simulink model "UNrobot_pro"  (R2021a)
settings: Solver=ode23t  StartTime=0.0  StopTime=t_end  FixedStep=dt  RelTol=1e-3
InitFcn:
  | RPInit
model workspace (MAT data in the model file):
  mapForSim.obsMap = [0 0 0 0 0 0 0 0 0 0 0 0 ... (40000 elements, 200x200)]
  mapForSim.scaleFactor = 5
  mapForSim.simMap = robotics.BinaryOccupancyGrid
  mapForSim.simMap.Grid = [1 1 1 1 1 1 1 1 1 1 1 1 ... (40000 elements, 200x200)]
  mapForSim.simMap.SharedProperties = matlabshared.autonomous.internal.SharedMapProperties
  mapForSim.simMap.SharedProperties.Resolution = 5
  mapForSim.simMap.SharedProperties.GridSize = [200 200]
  mapForSim.simMap.SharedProperties.XLocalLimits = [0 40]
  mapForSim.simMap.SharedProperties.YLocalLimits = [0 40]
  mapForSim.simMap.SharedProperties.XWorldLimits = [0 40]
  mapForSim.simMap.SharedProperties.YWorldLimits = [0 40]
  mapForSim.simMap.SharedProperties.Width = 40
  mapForSim.simMap.SharedProperties.Height = 40
  mapForSim.simMap.SharedProperties.LocalOriginInWorldInternal = [0 0]
  mapForSim.simMap.LayerName = 'binaryLayer'
  mapForSim.simMap.Index = matlabshared.autonomous.internal.CircularBufferIndex
  mapForSim.simMap.Index.Head = [1 1]
  mapForSim.simMap.Index.Size = [200 200]
  mapForSim.simMap.Index.NewRegions = [0 0 0 0]
  mapForSim.simMap.Index.DropEntireMap = 0
  mapForSim.simMap.Index.DropTwoRegions = [0 0]
  mapForSim.simMap.Buffer = matlabshared.autonomous.internal.CircularBuffer
  mapForSim.simMap.Buffer.ConstVal = 0
  mapForSim.simMap.Buffer.DataType = 'logical'
  mapForSim.simMap.Buffer.Index = matlabshared.autonomous.internal.CircularBufferIndex
  mapForSim.simMap.Buffer.Index.Head = [1 1]
  mapForSim.simMap.Buffer.Index.Size = [200 200]
  mapForSim.simMap.Buffer.Index.NewRegions = [0 0 0 0]
  mapForSim.simMap.Buffer.Index.DropEntireMap = 0
  mapForSim.simMap.Buffer.Index.DropTwoRegions = [0 0]
  mapForSim.simMap.Buffer.Buffer = [1 1 1 1 1 1 1 1 1 1 1 1 ... (40000 elements, 200x200)]
  mapForSim.simMap.Buffer.BufferSize = [200 200 1]
  mapForSim.simMap.DefaultValueInternal = 0
  mapForSim.simMap.DataSize = [200 200]
  mapForSim.simMap.GridLocationInWorld = [0 0]
  mapForSim.simMap.GridOriginInLocal = [0 0]
  mapForSim.simMap.LocalOriginInWorld = [0 0]
  mapForSim.simMap.Resolution = 5
  mapForSim.simMap.GridSize = [200 200]
  mapForSim.simMap.XLocalLimits = [0 40]
  mapForSim.simMap.YLocalLimits = [0 40]
  mapForSim.simMap.XWorldLimits = [0 40]
  mapForSim.simMap.YWorldLimits = [0 40]
  mapForSim.simMap.Width = 40
  mapForSim.simMap.Height = 40
  mapForSim.simMap.LocalOriginInWorldInternal = [0 0]
  occGrid = robotics.BinaryOccupancyGrid
  occGrid.Grid = [1 1 1 1 1 1 1 1 1 1 1 1 ... (40000 elements, 200x200)]
  occGrid.SharedProperties = matlabshared.autonomous.internal.SharedMapProperties
  occGrid.SharedProperties.Resolution = 5
  occGrid.SharedProperties.GridSize = [200 200]
  occGrid.SharedProperties.XLocalLimits = [0 40]
  occGrid.SharedProperties.YLocalLimits = [0 40]
  occGrid.SharedProperties.XWorldLimits = [0 40]
  occGrid.SharedProperties.YWorldLimits = [0 40]
  occGrid.SharedProperties.Width = 40
  occGrid.SharedProperties.Height = 40
  occGrid.SharedProperties.LocalOriginInWorldInternal = [0 0]
  occGrid.LayerName = 'binaryLayer'
  occGrid.Index = matlabshared.autonomous.internal.CircularBufferIndex
  occGrid.Index.Head = [1 1]
  occGrid.Index.Size = [200 200]
  occGrid.Index.NewRegions = [0 0 0 0]
  occGrid.Index.DropEntireMap = 0
  occGrid.Index.DropTwoRegions = [0 0]
  occGrid.Buffer = matlabshared.autonomous.internal.CircularBuffer
  occGrid.Buffer.ConstVal = 0
  occGrid.Buffer.DataType = 'logical'
  occGrid.Buffer.Index = matlabshared.autonomous.internal.CircularBufferIndex
  occGrid.Buffer.Index.Head = [1 1]
  occGrid.Buffer.Index.Size = [200 200]
  occGrid.Buffer.Index.NewRegions = [0 0 0 0]
  occGrid.Buffer.Index.DropEntireMap = 0
  occGrid.Buffer.Index.DropTwoRegions = [0 0]
  occGrid.Buffer.Buffer = [1 1 1 1 1 1 1 1 1 1 1 1 ... (40000 elements, 200x200)]
  occGrid.Buffer.BufferSize = [200 200 1]
  occGrid.DefaultValueInternal = 0
  occGrid.DataSize = [200 200]
  occGrid.GridLocationInWorld = [0 0]
  occGrid.GridOriginInLocal = [0 0]
  occGrid.LocalOriginInWorld = [0 0]
  occGrid.Resolution = 5
  occGrid.GridSize = [200 200]
  occGrid.XLocalLimits = [0 40]
  occGrid.YLocalLimits = [0 40]
  occGrid.XWorldLimits = [0 40]
  occGrid.YWorldLimits = [0 40]
  occGrid.Width = 40
  occGrid.Height = 40
  occGrid.LocalOriginInWorldInternal = [0 0]
values from neighbouring files (symbols this model uses):
  obstacles = eval(get_param(block,'obstacles'))    [RPInit.m]    (also in setup.m = csvread('obstacles2.csv'))
  Ts = 0.1    [setup.m]
undefined symbols (not defined in the file or in its folder): FloorSurface, Ref, RobotSurface, T_max, Wall1Surface, Wall2Surface, Wall3Surface, Wall4Surface, WallSurface, X, Y, Z
libraries: sm_lib x52, nesl_utility x18, RP_Simulator_Components x16, RoboticsPlayground x9, simulink x6
(part 1 of 3)
settings Model: EnablePacing=on  Creator=josea  LastModifiedBy=Sebastian
settings SolverCC: AlgebraicLoopSolver=TrustRegion
settings DataIOCC: ReturnWorkspaceOutputs=off
settings DebuggingCC: UnconnectedLineMsg=none  SFMachineParentedDataDiag=warning  ArithmeticOperatorsInVariantConditions=warning
settings SFSimCC: SimUseLocalCustomCode=off  CustomCodeUndefinedFunction=UseInterfaceOnly
settings RTWCC: RTWUseLocalCustomCode=off
settings DiagnosticsConfigSet: SimMechanicsRigidlyBoundBlock=none
settings ExplorerConfigSet: InternalSimMechanicsExplorerSettings="<ExplorerConfiguration><canonicalview>default</canonicalview><AnimationSetting><BasePlaybackSpeed>1.0</BasePlaybackSpeed><PlaybackSpeedFactor>1.0</PlaybackSpeedFactor></AnimationSetting><TilePanel><TileInfo><Tiles Columns=\"2\" Count=\"3\" Rows=\"2\"><Column Weight=\"0.4996\"/><Column Weight=\"0.5004\"/><Row Weight=\"0.4995\"/><Row Weight=\"0.5005\"/><Tile Height=\"1\" Width=\"2\" X=\"0\" Y=\"0\"/><Tile Height=\"1\" Width=\"1\" X=\"0\" Y=\"1\"/><Tile Height=\"1\" Width=\"1\" X=\"1\" Y=\"1\"/></Tiles></TileInfo><SceneInfo><SceneViewer><BGColor><R>0.400000005960464478</R><G>0.400000005960464478</G><B>0.400000005960464478</B></BGColor><Camera><DoPerspective>off</DoPerspective><Position><X>42.9310669159878344</X><Y>-10.3897658506810977</Y><Z>43.7453005085714111</Z></Position><Center><X>20.3419761828377759</X><Y>23.2650901944664916</Y><Z>12.1932033045180681</Z></Center><Up><X>-0.363361854461093647</X><Y>0.495671071722158407</Y><Z>0.788846215291930219</Z></Up><ViewLimDist>1</ViewLimDist><YLim>30.3164478917145566</YLim><XLim>117.138200069864226</XLim></Camera></SceneViewer><SceneViewer><BGColor><R>0.400000005960464478</R><G>0.400000005960464478</G><B>0.400000005960464478</B></BGColor><Camera><DoPerspective>on</DoPerspective><Position><X>8.06324715656376156</X><Y>-1.11711218962495051</Y><Z>0.353907143146574898</Z></Position><Center><X>7.7585532943741855</X><Y>-0.164661849531568261</Y><Z>0.353907143146574954</Z></Center><Up><X>5.06422372314121883e-17</X><Y>-4.83127509520006689e-17</Y><Z>1</Z></Up><ViewLimDist>1</ViewLimDist><YLim>0.466307658154998583</YLim><XLim>0.89330132171144927</XLim></Camera></SceneViewer><SceneViewer><BGColor><R>0.400000005960464478</R><G>0.400000005960464478</G><B>0.400000005960464478</B></BGColor><Camera><DoPerspective>off</DoPerspective><Position><X>9.39383108584540416</X><Y>-0.802378430868030179</Y><Z>41.4375460163895966</Z></Position><Center><X>9.39383108584540416</X><Y>-0.802378430868030179</Y><Z>2.33605756749020088</Z></Center><Up><X>0</X><Y>1</Y><Z>-0</Z></Up><ViewLimDist>1</ViewLimDist><YLim>18.9446942541944559</YLim><XLim>36.3365447170614928</XLim></Camera></SceneViewer></SceneInfo></TilePanel><MechEditorPanel><Cameras><Camera><Id>Camera1</Id><Value><Name>RobotView</Name><NativeCamera><PositionTrackingFeature>Obstacle_Environment.Robot.Body.RobotCamera.F</PositionTrackingFeature><CenterTrackingFeature>Obstacle_Environment.Robot.Body.RobotCamera.F</CenterTrackingFeature><UpVectorTrackingFeature>Obstacle_Environment.Robot.Body.RobotCamera.F</UpVectorTrackingFeature><CenterTrackingOrigin>off</CenterTrackingOrigin><CenterTrackingDirection>+X</CenterTrackingDirection><UpVectorTrackingDirection>+Z</UpVectorTrackingDirection></NativeCamera></Value></Camera></Cameras><GfxPanelCameraMap><MapElement CameraMLId=\"Camera1\" GfxPanelIndex=\"1\"/></GfxPanelCameraMap><VideoCreator><PlaybackSpeedRatio>1.0</PlaybackSpeedRatio><FrameRate>30</FrameRate><VideoFormat>MPEG-4</VideoFormat><FrameSize>[1920 1080]</FrameSize></VideoCreator></MechEditorPanel></ExplorerConfiguration>"

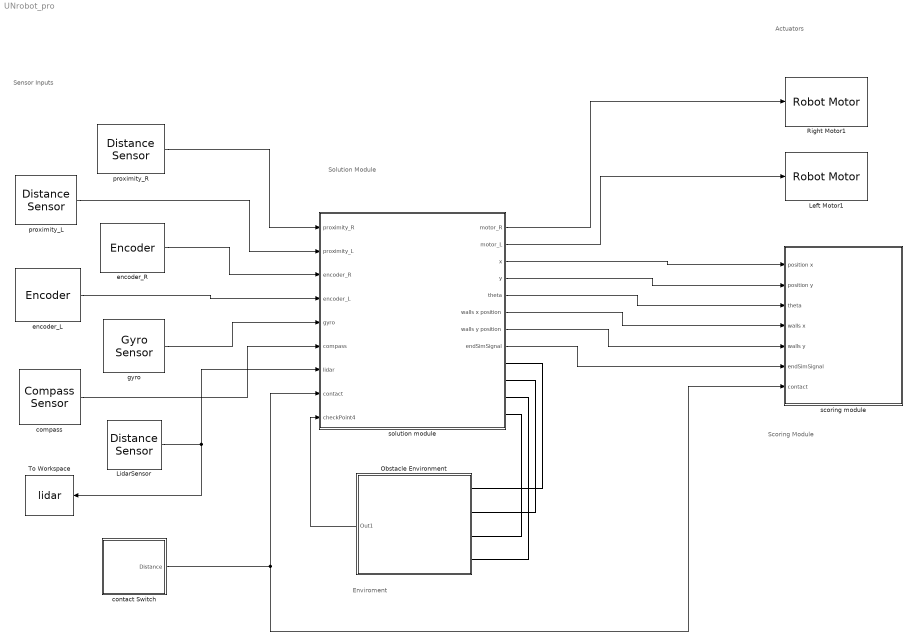
== system UNrobot_pro ==
  note: Solution Module
  note: Actuators
  note: Scoring Module
  note: Sensor Inputs
  note: Enviroment
  Left Motor1 : RoboticsPlayground/Basic Sensors and Actuators/Robot Motor  robotId=1  motorChoice=1
      settings: SourceProductName=Robotics Playground
  LidarSensor : RoboticsPlayground/Basic Sensors and Actuators/Distance Sensor  robotId=1  maxSenRange=4  minSenRange=0.02  senRes=0.01  sensOff=[-0.1 0]  sensOffDeg=0  sensorTs=0.1  mask(RP Distance Sensor){}
      link override MATLAB System: scanAngles=linspace(-pi,pi,37)
      settings: SourceProductName=Robotics Playground
      mask Display: image('$imagefile'); % Use "Edit Image" on toolstrip to change.
  Obstacle Environment : Subsystem  mask(RP Obstacle Environment){obstacles=obstacles, arenaLength=40, arenaWidth=40, robotId=1, wheelBase=0.5, wheelRadius=0.1, robotColor=[0.5 0 0], startPose=[0 0]}
      mask prompts: obstacles "Obstacles matrix[nx4] with rectangles with the form [x,y,length,width]"; arenaLength "Length [m]"; arenaWidth "Width [m]"; robotId "Robot ID"; wheelBase "Distance between wheels [m]"; wheelRadius "Wheel radius [m]"; robotColor "Color [R G B]"; startPose "Initial Position X Y [m]"
      mask help:
      | This block contains a virtual environment for a single robot to interact with walls, obstacles and objects. Sensors implemented in the Robotics Playground library can be used to obtain environment information and actuators to interact with the robot behavior.
      |
      | Motor mapping for the robot is as follows:
      |
      | Motor 1 -> Left wheel motor torque
      | Motor 2 -> Right wheel motor torque
      settings: CopyFcn=|
      | set_param(gcs,'InitFcn','RPInit');
      | set_param(gcs,'Solver','ode23t');
      | set_param(gcs, 'EnablePacing', 'on')
      | set_param(gcs, 'PacingRate', 1)
      mask Help: web('obstacle_arena.htm')
      mask DialogControl obsT Prompt: Obstacle settings
      mask DialogControl Container19 Prompt: Set Obstacles Interactively
      mask DialogControl Control2 Prompt: Set Obstacles
      mask DialogControl Control2 Callback: setObstaclesUI(gcb)
      mask DialogControl Container6 Prompt: Arena settings
      mask DialogControl Container4 Prompt: Robot settings
      mask Display:
      | color('white');
      | plot([100,100,100,100]*1,[100,100,100,100]*1);
      | plot([100,100,100,100]*0,[100,100,100,100]*0);
      | image('ObstacleEnv.PNG')
      | color('blue');
      | id=eval(get_param(gcb,'robotId'));
      | text(99, 92, ['Robot ID: ' num2str(id)], 'horizontalAlignment', 'right');
  Right Motor1 : RoboticsPlayground/Basic Sensors and Actuators/Robot Motor  robotId=1  motorChoice=2
      settings: SourceProductName=Robotics Playground
  To Workspace : ToWorkspace  VariableName=lidar  SaveFormat=Structure  SampleTime=-1
  "compass " : RoboticsPlayground/Basic Sensors and Actuators/Compass Sensor  robotId=1  sensorTs=0.01
      settings: SourceProductName=Robotics Playground
  contact Switch : Subsystem  AncestorBlock=RoboticsPlayground/Basic Sensors and Actuators/Contact Switch  mask(RP Contact Switch){robotId=1, trigDist=0.251, sensOff=[0 0], sensOffDeg=0, sensorTs=0.1}
      mask prompts: robotId "Robot ID"; trigDist "Trigger Distance [m]"; sensOff "Sensor Position Offset X Y [m]"; sensOffDeg "Sensor Orientation Offset [deg]"; sensorTs "Sensor sample time [s]"
      mask help:
      | This block outputs 1 if the sensor comes in close proximity to a wall or obstacle. Otherwise it outputs zero. The proximity at which the sensor is triggered can be set through the mask using the "Trigger Distance" field. Default values can also be used.
      |
      | Sensor position and orientation offsets are with respect to the robot center.
      mask init:
      | ID=get_param(gcb,'robotId');
      | 
      | set_param([gcb '/xPose'],'GotoTag',['R' ID 'xPose']);
      | set_param([gcb '/yPose'],'GotoTag',['R' ID 'yPose']);
      | set_param([gcb '/tPose'],'GotoTag',['R' ID 'tPose']);
      mask Help: web('contact_switch.htm')
      mask DialogControl senCont Prompt: Sensor Characteristics
      mask Display:
      | color('white');
      | plot([100,100,100,100]*1,[100,100,100,100]*1);
      | plot([100,100,100,100]*0,[100,100,100,100]*0);
      | image('ContactSwitch.png','center')
      | color('blue');
      | id=eval(get_param(gcb,'robotId'));
      | text(99, 92, ['Robot ID: ' num2str(id)], 'horizontalAlignment', 'right');
  encoder_L : RoboticsPlayground/Basic Sensors and Actuators/Encoder  robotId=1  motorChoice=1  rstChoice=No reset  ticks=encoder_ticks  detectDir=on  sensorTs=0.1
      settings: SourceProductName=Robotics Playground
  encoder_R : RoboticsPlayground/Basic Sensors and Actuators/Encoder  robotId=1  motorChoice=2  rstChoice=No reset  ticks=encoder_ticks  detectDir=on  sensorTs=0.1
      settings: SourceProductName=Robotics Playground
  "gyro " : RoboticsPlayground/Basic Sensors and Actuators/Gyro Sensor  robotId=1  sensor=Body Center  sensorTs=0.01
      settings: SourceProductName=Robotics Playground
  proximity_L : RoboticsPlayground/Basic Sensors and Actuators/Distance Sensor  robotId=1  maxSenRange=2  minSenRange=0.02  senRes=0.01  sensOff=P_L  sensOffDeg=45  sensorTs=0.1
      settings: SourceProductName=Robotics Playground
  proximity_R : RoboticsPlayground/Basic Sensors and Actuators/Distance Sensor  robotId=1  maxSenRange=2  minSenRange=0.02  senRes=0.01  sensOff=P_R  sensOffDeg=-45  sensorTs=0.1  mask(RP Distance Sensor){}
      settings: SourceProductName=Robotics Playground
  scoring module : Subsystem
  solution module : Subsystem
  wires:
  proximity_R/1 -> solution module/1(proximity_R)
  proximity_L/1 -> solution module/2(proximity_L)
  encoder_R/1 -> solution module/3(encoder_R)
  encoder_L/1 -> solution module/4(encoder_L)
  "gyro "/1 -> solution module/5(gyro)
  "compass "/1 -> solution module/6(compass)
  contact Switch/1(Distance) -> solution module/8(contact), scoring module/7(contact)
  solution module/2(motor_L) -> Left Motor1/1
  solution module/1(motor_R) -> Right Motor1/1
  solution module/3(x) -> scoring module/1(position x)
  solution module/4(y) -> scoring module/2(position y)
  solution module/5(theta) -> scoring module/3(theta)
  Obstacle Environment/1(Out1) -> solution module/9(checkPoint4)
  LidarSensor/1 -> To Workspace/1, solution module/7(lidar)
  solution module/6(walls x position) -> scoring module/4(walls x)
  solution module/7(walls y position) -> scoring module/5(walls y)
  solution module/8(endSimSignal) -> scoring module/6(endSimSignal)
  connections:
  Obstacle Environment/LConn4 -- solution module/RConn3
  Obstacle Environment/LConn1 -- solution module/RConn1
  Obstacle Environment/LConn2 -- solution module/RConn2
  Obstacle Environment/LConn3 -- solution module/RConn4

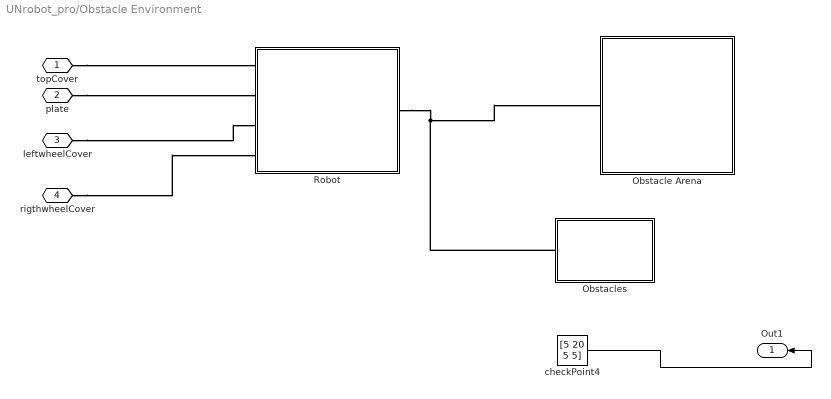
== system UNrobot_pro/Obstacle Environment ==
  Obstacle Arena : Subsystem  AncestorBlock=RP_Simulator_Components/Obstacle Arena  mask(RP Grid Arena){length=arenaLength, width=arenaWidth, robotRadius=wheelBase/2, checkPoint4=[5 20 5 5]}
      mask prompts: length "Arena length [m]"; width "Arena width [m]"; robotRadius "Robot Radius [m]"; checkPoint4 "check point 4 position [x,y, Length Width]"
      mask help: This block is an arena for robots to operate within. This arena implements contact between one robot and the walls and also introduces a floor grid for better visualization. Connect to other robots within the library using the corresponding "Robot" and "Ref" ports.
      mask DialogControl Container5 Prompt: Arena dimensions
      mask Display:
      | image('ObstacleArena.PNG')
      | port_label('Lconn',1,'RP-Bus')
  Obstacles : Subsystem
  Robot : Subsystem  AncestorBlock=RP_Simulator_Components/Contact Tank Robot  mask(RP Contact Tank Robot){robotId=robotId, wheelRadius=wheelRadius, wheelBase=wheelBase, wheelThickness=0.025, chassisThickness=0.05, startPose=startPose, choice=off, sensorTs=0.05, wheelMass=0.2, chassisMass=0.5, maxWheelTorque=T_max, floorSize=[arenaLength arenaWidth], wheelColor=[0.25 0.25 0.25], chassisColor=robotColor}
      mask prompts: robotId "Robot ID"; wheelRadius "Wheel Radius [m]"; wheelBase "Wheelbase [m]"; wheelThickness "Wheel Thickness [m]"; chassisThickness "Chassis Thickness [m]"; startPose "Start Position [m]"; choice "Reverse Start Position"; sensorTs "Sensor sample time [s]"; wheelMass "Wheel Mass [kg]"; chassisMass "Chassis Mass [kg]"; maxWheelTorque "Maximum wheel torque [N*m]"; floorSize "Floor Dimensions [m]"; wheelColor "Wheel Color"; chassisColor "Chassis Color"
      mask help:
      | This robot implements contact between the robot wheels and the floor of an arena. The stck-slip friction implemented using contact force libraries makes the robot behavior more realistic. The inputs to the robot are now motor torque, which is set using the Robotics Playground Motor blocks. The motor mappings are as follows:
      |
      | Motor 1 -> Left wheel motor torque
      | Motor 2 -> Right wheel motor torque
      mask init:
      | block=gcb;
      | ID=num2str(eval(get_param(block,'robotId')));
      | 
      | set_param([block '/motor1t'],'GotoTag',['R' ID 'motor1t']);
      | set_param([block '/motor2t'],'GotoTag',['R' ID 'motor2t']);
      | set_param([block '/motor1q'],'GotoTag',['R' ID 'motor1q']);
      | set_param([block '/motor1w'],'GotoTag',['R' ID 'motor1w']);
      | set_param([block '/motor2q'],'GotoTag',['R' ID 'motor2q']);
      | set_param([block '/motor2w'],'GotoTag',['R' ID 'motor2w']);
      | set_param([block '/xPose'],'GotoTag',['R' ID 'xPose']);
      | set_param([block '/yPose'],'GotoTag',['R' ID 'yPose']);
      | set_param([block '/tPose'],'GotoTag',['R' ID 'tPose']);
      | set_param([block '/tRate'],'GotoTag',['R' ID 'tRate']);
      | set_param([block '/tAngle'],'GotoTag',['R' ID 'tAngle']);
      | 
      | % Add sensor visuals
      | 
      | addSensors(block,eval(ID));
      mask DialogControl KinContainer Prompt: Kinematics
      mask DialogControl DynamicsContainer Prompt: Dynamics
      mask DialogControl AppearanceContainer Prompt: Appearance
      mask Display:
      | image('discRobot.PNG')
      | port_label('Rconn',1,'RP-Bus')
  checkPoint4 : Constant  Value=[5 20 5 5]
  topCover : PMIOPort  Side=Left
  plate : PMIOPort  Port=2  Side=Left
  leftwheelCover : PMIOPort  Port=3  Side=Left
  rigthwheelCover : PMIOPort  Port=4  Side=Left
  Out1 : Outport
  wires:
  checkPoint4/1 -> Out1/1
  connections:
  Obstacles/LConn1 -- Robot/RConn1 -- Obstacle Arena/LConn1
  topCover/RConn1 -- Robot/LConn1
  plate/RConn1 -- Robot/LConn2
  leftwheelCover/RConn1 -- Robot/LConn3
  rigthwheelCover/RConn1 -- Robot/LConn4

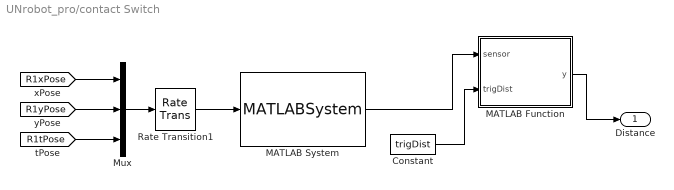
== system UNrobot_pro/contact Switch ==
  Constant : Constant  Value=trigDist
  MATLAB Function : MATLAB Function  TreatAsAtomicUnit=on
  MATLAB System : MATLABSystem  System=LidarSensorRP  mapName=occGrid  sensorOffset=sensOff  scanAngles=linspace(-pi,pi,50)  maxRange=trigDist+1
      mask Type: LidarSensorRP
      mask Display:
      | disp(['Lidar' char(10) 'Sensor']);
      | port_label('input',1,'pose');
      | port_label('output',1,'ranges');
  Mux : Mux  Inputs=3
  Rate Transition1 : RateTransition  OutPortSampleTime=sensorTs
  Distance : Outport  VectorParamsAs1DForOutWhenUnconnected=off
  wires:
  Rate Transition1/1 -> MATLAB System/1
  MATLAB Function/1(y) -> Distance/1
  Constant/1 -> MATLAB Function/2(trigDist)
  MATLAB System/1 -> MATLAB Function/1(sensor)
  [R1xPose] -> Mux/1
  [R1yPose] -> Mux/2
  [R1tPose] -> Mux/3
  Mux/1 -> Rate Transition1/1

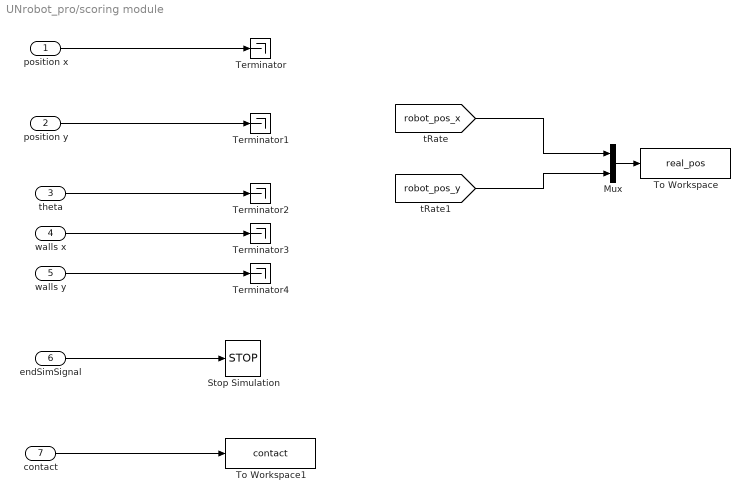
== system UNrobot_pro/scoring module ==
  position x : Inport
  position y : Inport  Port=2
  theta : Inport  Port=3
  walls x : Inport  Port=4
  walls y : Inport  Port=5
  endSimSignal : Inport  Port=6
  contact : Inport  Port=7
  Mux : Mux  Inputs=2
  Stop Simulation : Stop
  Terminator{,1..4} (5 alike) : Terminator
  To Workspace : ToWorkspace  VariableName=real_pos  SaveFormat=Structure With Time  SampleTime=Ts
  To Workspace1 : ToWorkspace  VariableName=contact  SaveFormat=Structure  SampleTime=Ts
  wires:
  position x/1 -> Terminator/1
  position y/1 -> Terminator1/1
  theta/1 -> Terminator2/1
  [robot_pos_x] -> Mux/1
  [robot_pos_y] -> Mux/2
  Mux/1 -> To Workspace/1
  endSimSignal/1 -> Stop Simulation/1
  contact/1 -> To Workspace1/1
  walls x/1 -> Terminator3/1
  walls y/1 -> Terminator4/1

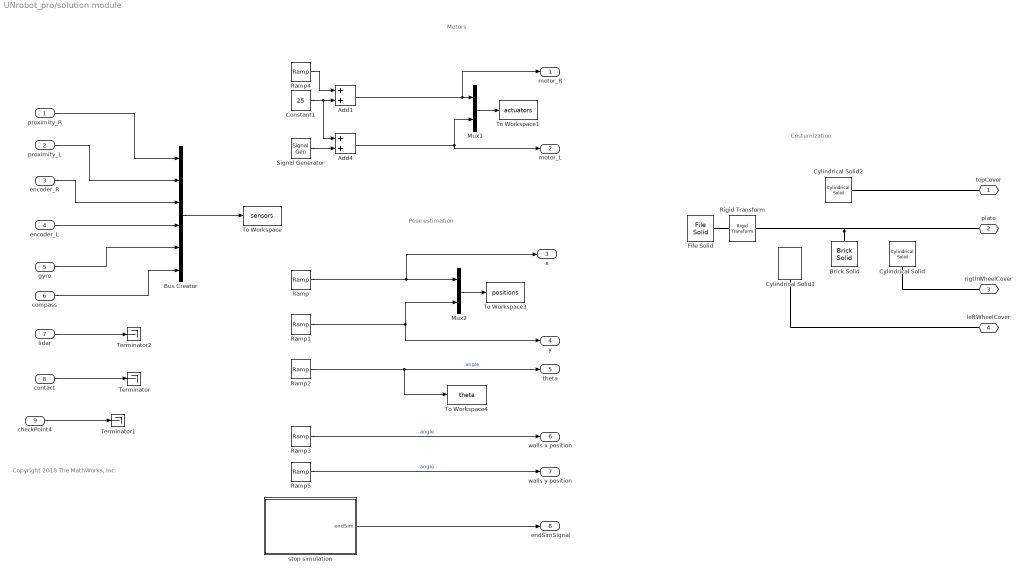
== system UNrobot_pro/solution module ==
  note: Copyright 2018 The MathWorks, Inc.
  note: Pose estimation
  note: Costumization
  note: Motors
  proximity_R : Inport
  proximity_L : Inport  Port=2
  encoder_R : Inport  Port=3
  encoder_L : Inport  Port=4
  gyro : Inport  Port=5
  compass : Inport  Port=6
  lidar : Inport  Port=7
  contact : Inport  Port=8
  checkPoint4 : Inport  Port=9
  Add1 : Sum
  Add4 : Sum
  Brick Solid : sm_lib/Body Elements/Brick Solid  GraphicAmbientColor=[0.15 0.15 0.15 1.0]  BasedOnType=Density  BrickDimensions=[0.1 0.25 0.05]  BrickDimensionUnits=m  CenterOfMass=[0 0 0]  CenterOfMassUnits=m  GraphicDiffuseColor=[ 0 1 0.5]  Density=1000  DensityUnits=kg/m^3  DoExposeReferenceFrame=off  GraphicEmissiveColor=[0.0 0.0 0.0 1.0]  ExportEntireGeometry=off  SerializedFrames=<Frames><Frame><Id>Frame1</Id><Value><Name>F1</Name><Origin><Source>GeometricFeature</Source><FeatureName>+z surface</FeatureName></Origin><PrimaryAxis><DefinedDirection>+Z</DefinedDirection><Source>ReferenceFrame</Source><SourceDirection>+Z</SourceDirection><FeatureName></FeatureName></PrimaryAxis><SecondaryAxis><DefinedDirection>+X</DefinedDirection><Source>ReferenceFrame</Source><SourceDirection>+X</SourceDirection><FeatureName></FeatureName></SecondaryAxis></Value></Frame></Frames>  MarkerShape=Sphere  MarkerSize=10  GraphicType=FromGeometry  InertiaType=PointMass  Mass=0  MassUnits=kg  MomentsOfInertia=[1 1 1]  MomentsOfInertiaUnits=kg*m^2  GraphicOpacity=0.4  ProductsOfInertia=[0 0 0]  ProductsOfInertiaUnits=kg*m^2  GraphicShininess=75  GraphicSpecularColor=[0.5 0.5 0.5 1.0]  GraphicVisPropType=SimpleVisualProperties
  Bus Creator : BusCreator  Inputs=6
  Constant1 : Constant  Value=25
  Cylindrical Solid : sm_lib/Body Elements/Cylindrical Solid  GraphicAmbientColor=[0.15 0.15 0.15 1.0]  BasedOnType=Density  CenterOfMass=[0 0 0]  CenterOfMassUnits=m  GraphicDiffuseColor=[0 1 0.5]  CylinderLength=0.05  CylinderLengthUnits=m  CylinderRadius=0.1  CylinderRadiusUnits=m  Density=1000  DensityUnits=kg/m^3  DoExposeReferenceFrame=off  GraphicEmissiveColor=[0.0 0.0 0.0 1.0]  ExportEntireGeometry=off  SerializedFrames=<Frames><Frame><Id>Frame1</Id><Value><Name>F1</Name><Origin><Source>GeometricFeature</Source><FeatureName>bottom surface</FeatureName></Origin><PrimaryAxis><DefinedDirection>+Z</DefinedDirection><Source>ReferenceFrame</Source><SourceDirection>+Z</SourceDirection><FeatureName></FeatureName></PrimaryAxis><SecondaryAxis><DefinedDirection>+X</DefinedDirection><Source>ReferenceFrame</Source><SourceDirection>+X</SourceDirection><FeatureName></FeatureName></SecondaryAxis></Value></Frame></Frames>  MarkerShape=Sphere  MarkerSize=10  GraphicType=FromGeometry  InertiaType=CalculateFromGeometry  Mass=1  MassUnits=kg  MomentsOfInertia=[1 1 1]  MomentsOfInertiaUnits=kg*m^2  GraphicOpacity=0.1  ProductsOfInertia=[0 0 0]  ProductsOfInertiaUnits=kg*m^2  GraphicShininess=75  GraphicSpecularColor=[0.5 0.5 0.5 1.0]  GraphicVisPropType=SimpleVisualProperties
  Cylindrical Solid1 : sm_lib/Body Elements/Cylindrical Solid  GraphicAmbientColor=[0.15 0.15 0.15 1.0]  BasedOnType=Density  CenterOfMass=[0 0 0]  CenterOfMassUnits=m  GraphicDiffuseColor=[0 1 0.5 ]  CylinderLength=0.05  CylinderLengthUnits=m  CylinderRadius=0.1  CylinderRadiusUnits=m  Density=1000  DensityUnits=kg/m^3  DoExposeReferenceFrame=off  GraphicEmissiveColor=[0.0 0.0 0.0 1.0]  ExportEntireGeometry=off  SerializedFrames=<Frames><Frame><Id>Frame1</Id><Value><Name>F1</Name><Origin><Source>GeometricFeature</Source><FeatureName>bottom surface</FeatureName></Origin><PrimaryAxis><DefinedDirection>+Z</DefinedDirection><Source>ReferenceFrame</Source><SourceDirection>+Z</SourceDirection><FeatureName></FeatureName></PrimaryAxis><SecondaryAxis><DefinedDirection>+X</DefinedDirection><Source>ReferenceFrame</Source><SourceDirection>+X</SourceDirection><FeatureName></FeatureName></SecondaryAxis></Value></Frame></Frames>  MarkerShape=Sphere  MarkerSize=10  GraphicType=FromGeometry  InertiaType=PointMass  Mass=0  MassUnits=kg  MomentsOfInertia=[1 1 1]  MomentsOfInertiaUnits=kg*m^2  GraphicOpacity=0.1  ProductsOfInertia=[0 0 0]  ProductsOfInertiaUnits=kg*m^2  GraphicShininess=75  GraphicSpecularColor=[0.5 0.5 0.5 1.0]  GraphicVisPropType=SimpleVisualProperties
  Cylindrical Solid2 : sm_lib/Body Elements/Cylindrical Solid  GraphicAmbientColor=[0.15 0.15 0.15 1.0]  BasedOnType=Density  CenterOfMass=[0 0 0]  CenterOfMassUnits=m  GraphicDiffuseColor=[0 1 0.5]  CylinderLength=0.5  CylinderLengthUnits=m  CylinderRadius=0.25  CylinderRadiusUnits=m  Density=1000  DensityUnits=kg/m^3  DoExposeReferenceFrame=off  GraphicEmissiveColor=[0.0 0.0 0.0 1.0]  ExportEntireGeometry=off  SerializedFrames=<Frames><Frame><Id>Frame1</Id><Value><Name>F1</Name><Origin><Source>GeometricFeature</Source><FeatureName>bottom surface</FeatureName></Origin><PrimaryAxis><DefinedDirection>+Z</DefinedDirection><Source>ReferenceFrame</Source><SourceDirection>+Z</SourceDirection><FeatureName></FeatureName></PrimaryAxis><SecondaryAxis><DefinedDirection>+X</DefinedDirection><Source>ReferenceFrame</Source><SourceDirection>+X</SourceDirection><FeatureName></FeatureName></SecondaryAxis></Value></Frame></Frames>  MarkerShape=Sphere  MarkerSize=10  GraphicType=FromGeometry  InertiaType=PointMass  Mass=0  MassUnits=kg  MomentsOfInertia=[1 1 1]  MomentsOfInertiaUnits=kg*m^2  GraphicOpacity=0.1  ProductsOfInertia=[0 0 0]  ProductsOfInertiaUnits=kg*m^2  GraphicShininess=75  GraphicSpecularColor=[0.5 0.5 0.5 1.0]  GraphicVisPropType=SimpleVisualProperties
  File Solid : sm_lib/Body Elements/File Solid  ExtGeomFileName=CAD\placa.step  UnitType=FromFile  ExtGeomFileUnits=cm  StepReaderType=HEX  ExportConvexHullGeometry=off  InertiaType=PointMass  Mass=0  MassUnits=kg  CenterOfMass=[0 0 0]  CenterOfMassUnits=m  MomentsOfInertia=[1 1 1]  MomentsOfInertiaUnits=kg*m^2  ProductsOfInertia=[0 0 0]  ProductsOfInertiaUnits=kg*m^2  BasedOnType=DensityFromFile  Density=1000  DensityUnits=kg/m^3  DoExposeReferenceFrame=on  SerializedFrames=<Frames/>  GraphicType=FromGeometry  MarkerShape=Sphere  MarkerSize=10  GraphicVisPropType=SimpleVisualProperties  GraphicDiffuseColor=[1 1 1]  GraphicSpecularColor=[0.5 0.5 0.5 1.0]  GraphicAmbientColor=[0.15 0.15 0.15 1.0]  GraphicEmissiveColor=[0.0 0.0 0.0 1.0]  GraphicShininess=75  GraphicOpacity=1.0
  Mux1 : Mux  Inputs=2
  Mux2 : Mux  Inputs=2
  Ramp{,1..5} (6 alike) : simulink/Sources/Ramp  slope=1  start=0  InitialOutput=0
  Rigid Transform : sm_lib/Frames and Transforms/Rigid Transform  TranslationMethod=None  TranslationStandardOffset=0  TranslationLengthUnit=m  TranslationStandardAxis=+Z  TranslationCartesianOffset=[0 0 0]  TranslationROffset=0  TranslationROffsetUnits=m  TranslationZOffset=0  TranslationZOffsetUnits=m  TranslationThetaOffset=0  TranslationThetaOffsetUnits=deg  RotationMethod=RotationSequence  RotationAngleUnits=deg  RotationStandardAxis=+Z  RotationAngle=0.0  RotationArbitraryAxis=[0 0 1]  FollAlignAxisA=+X  BaseAlignAxisA=+Y  FollAlignAxisB=+Y  BaseAlignAxisB=+Z  RotationSequenceAxes=FollowerAxes  RotationSequence=YXZ  RotationSequenceAngles=[180 0 0]  RotationSequenceAnglesUnits=deg  RotationMatrix=[1 0 0; 0 1 0; 0 0 1]
  Signal Generator : SignalGenerator  WaveForm=sawtooth  Amplitude=10  Frequency=3  Units=rad/sec
  Terminator : Terminator
  Terminator1 : Terminator
  Terminator2 : Terminator
  To Workspace : ToWorkspace  VariableName=sensors  SaveFormat=Structure With Time  SampleTime=Ts
  To Workspace1 : ToWorkspace  VariableName=actuators  SaveFormat=Structure With Time  SampleTime=Ts
  To Workspace3 : ToWorkspace  VariableName=positions  SaveFormat=Structure With Time  SampleTime=Ts
  To Workspace4 : ToWorkspace  VariableName=theta  SaveFormat=Structure With Time  SampleTime=Ts
  stop simulation : Stateflow chart  TreatAsAtomicUnit=on
  topCover : PMIOPort  Side=Right
  plate : PMIOPort  Port=2  Side=Right
  rigthWheelCover : PMIOPort  Port=3  Side=Right
  leftWheelCover : PMIOPort  Port=4  Side=Right
  motor_R : Outport
  motor_L : Outport  Port=2
  x : Outport  Port=3
  y : Outport  Port=4
  theta : Outport  Port=5
  walls x position : Outport  Port=6
  walls y position : Outport  Port=7
  endSimSignal : Outport  Port=8
  wires:
  checkPoint4/1 -> Terminator1/1
  lidar/1 -> Terminator2/1
  encoder_R/1 -> Bus Creator/3
  gyro/1 -> Bus Creator/5
  compass/1 -> Bus Creator/6
  proximity_L/1 -> Bus Creator/2
  Bus Creator/1 -> To Workspace/1
  encoder_L/1 -> Bus Creator/4
  proximity_R/1 -> Bus Creator/1
  contact/1 -> Terminator/1
  Ramp1/1 -> Mux2/2, y/1
  Ramp/1 -> x/1, Mux2/1
  Add4/1 -> Mux1/2, motor_L/1
  stop simulation/1(endSim) -> endSimSignal/1
  Mux2/1 -> To Workspace3/1
  Add1/1 -> motor_R/1, Mux1/1
  Ramp2/1 -> To Workspace4/1, theta/1  "angle"
  Constant1/1 -> Add1/2, Add4/1
  Ramp4/1 -> Add1/1
  Signal Generator/1 -> Add4/2
  Mux1/1 -> To Workspace1/1
  Ramp5/1 -> walls y position/1  "angle"
  Ramp3/1 -> walls x position/1  "angle"
  connections:
  Brick Solid/LConn1 -- Rigid Transform/LConn1 -- plate/RConn1
  File Solid/RConn1 -- Rigid Transform/RConn1
  Cylindrical Solid/LConn1 -- rigthWheelCover/RConn1
  Cylindrical Solid2/LConn1 -- topCover/RConn1
  Cylindrical Solid1/LConn1 -- leftWheelCover/RConn1

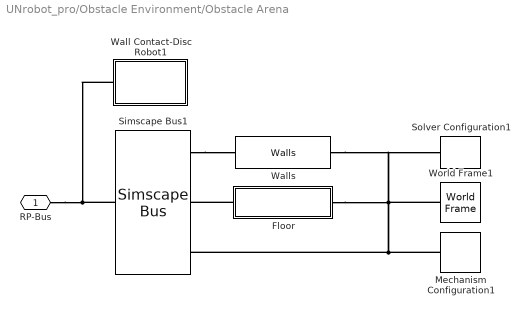
== system UNrobot_pro/Obstacle Environment/Obstacle Arena ==
  Floor : Subsystem  mask{checkPoint4=checkPoint4}
  Mechanism Configuration1 : sm_lib/Utilities/Mechanism Configuration  UniformGravity=Constant  GravityVector=[0 0 -9.80665]  GravityVectorUnits=m/s^2  GravityUnits=m/s^2  LinearizationDelta=0.001  JointModeTransitionNonlinearIterations=2
  Simscape Bus1 : SimscapeBus  HierarchyStrings=WallSurface;FloorSurface;Ref
  Solver Configuration1 : nesl_utility/Solver Configuration  PhysicalDomain=network_engine_domain  SubClassName=solver  LeftPortType=input  RightPortType=generic  Tones=[]  Harmonics=[]  SimulateNoise=off  Profile=off  UseLocalSampling=off  EnableSwitchedLinearOptims=on  FrequencyDomain=off  UseCCode=off  RelTol=0.001  AbsTol=1e-06  MinStep=1e-09  ToWorkspace=off  RevertToSquareIcSolve=off  NumHomotopyIterations=100  PhasorMode=off  PhasorModeNumHarmonics=1  DoDC=off  ResidualTolerance=1e-09  UseLocalSolver=off  LocalSolverChoice=NE_BACKWARD_EULER_ADVANCER  LocalSolverSampleTime=0.0002  DoFixedCost=off  MaxNonlinIter=10  MaxModeIter=2  ComputeImpulses=off  ImpulseIterations=2  LinearAlgebra=Sparse  EquationFormulation=NE_TIME_EF  DelaysMemoryBudget=1024  AutomaticFiltering=off  FilteringTimeConstant=0.001  PartitionStorageMethod=AS_NEEDED  PartitionMemoryBudget=1024  PartitionMethod=FAST
  Wall Contact-Disc Robot1 : Subsystem  AncestorBlock=RP_Simulator_Components/Wall Contact-Disc Robot  mask(RP Disc-Walls){length=length, width=width, height=0.3}
      mask prompts: length "Arena length [m]"; width "Arena width [m]"; height "Wall height [m] (Visual only)"
      mask help: This block introduces the walls visualizations to the environment along with the respective contact forces implementation for a disc robot.
      mask Display:
      | image('wallContactDisc.png')
      | port_label('Lconn',1,'RP-Bus')
  Walls : RP_Simulator_Components/Object Arena/Walls  length=length  width=width  height=0.3
  World Frame1 : sm_lib/Frames and Transforms/World Frame
  RP-Bus : PMIOPort  Side=Left
  connections:
  Simscape Bus1/LConn1 -- Walls/LConn1
  Floor/LConn1 -- Simscape Bus1/LConn2
  Mechanism Configuration1/RConn1 -- Simscape Bus1/LConn3 -- Walls/RConn1 -- Solver Configuration1/RConn1 -- Floor/RConn1 -- World Frame1/RConn1
  Simscape Bus1/RConn1 -- RP-Bus/RConn1 -- Wall Contact-Disc Robot1/LConn1

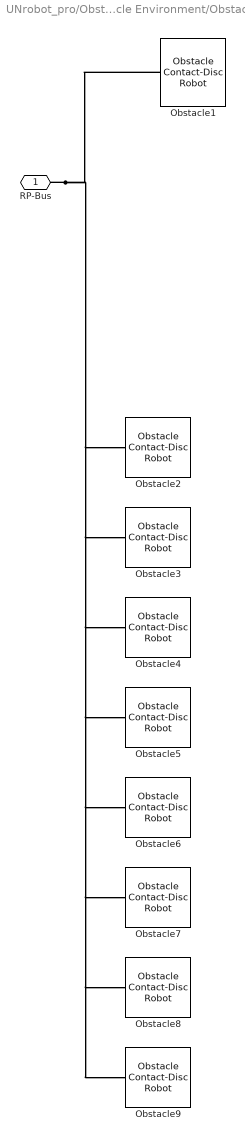
== system UNrobot_pro/Obstacle Environment/Obstacles ==
  Obstacle1 : RP_Simulator_Components/Obstacle Contact-Disc Robot  Pose=[2.55 -2.02]  width=1.96  length=9.1  height=0.3  color=[1.0 0.4 0.2]
      link override Solid: BrickDimensions=[length width height]
  Obstacle2 : RP_Simulator_Components/Obstacle Contact-Disc Robot  Pose=[8.01 -0.135000000000002]  width=5.55  length=1.94  height=0.3  color=[1.0 0.4 0.2]
      link override Solid: BrickDimensions=[length width height]
  Obstacle3 : RP_Simulator_Components/Obstacle Contact-Disc Robot  Pose=[12.51 1.405]  width=1.83  length=5.88  height=0.3  color=[1.0 0.4 0.2]
      link override Solid: BrickDimensions=[length width height]
  Obstacle4 : RP_Simulator_Components/Obstacle Contact-Disc Robot  Pose=[16.01 -3.9]  width=6  length=1.56  height=0.3  color=[1.0 0.4 0.2]
      link override Solid: BrickDimensions=[length width height]
  Obstacle5 : RP_Simulator_Components/Obstacle Contact-Disc Robot  Pose=[12.75 -7.845]  width=1.99  length=3.56  height=0.3  color=[1.0 0.4 0.2]
      link override Solid: BrickDimensions=[length width height]
  Obstacle6 : RP_Simulator_Components/Obstacle Contact-Disc Robot  Pose=[-3.39 2.78]  width=11.16  length=2.86  height=0.3  color=[1.0 0.4 0.2]
      link override Solid: BrickDimensions=[length width height]
  Obstacle7 : RP_Simulator_Components/Obstacle Contact-Disc Robot  Pose=[2.105 12.21]  width=1.56  length=14.39  height=0.3  color=[1.0 0.4 0.2]
      link override Solid: BrickDimensions=[length width height]
  Obstacle8 : RP_Simulator_Components/Obstacle Contact-Disc Robot  Pose=[10.24 13.615]  width=5.23  length=1.24  height=0.3  color=[1.0 0.4 0.2]
      link override Solid: BrickDimensions=[length width height]
  Obstacle9 : RP_Simulator_Components/Obstacle Contact-Disc Robot  Pose=[14.525 14.8]  width=1.02  length=6.79  height=0.3  color=[1.0 0.4 0.2]
      link override Solid: BrickDimensions=[length width height]
  RP-Bus : PMIOPort  Side=Left
  connections:
  Obstacle1/LConn1 -- Obstacle2/LConn1 -- Obstacle3/LConn1 -- Obstacle4/LConn1 -- Obstacle5/LConn1 -- Obstacle6/LConn1 -- Obstacle7/LConn1 -- Obstacle8/LConn1 -- RP-Bus/RConn1 -- Obstacle9/LConn1
